simulink model "Crtl_Model_SS"  (R2015a)
settings: Solver=ode45  StartTime=0.0  StopTime=10.0  RelTol=1e-3
values from neighbouring files (symbols this model uses):
  ssDot = n4sid(data33, 3, 'DisturbanceModel', 'none', Options)    [Model_Centralizat.m]
  ssTHPS = ss(ssTHPS)    [Model_Centralizat.m]
  Te = t(2)-t(1)    [Models.m]    (also in shit_try.m = 0.003; simData_check.mat = 0.01; smth_new_025.m)
settings Model: Creator=Maria  LastModifiedBy=Maria

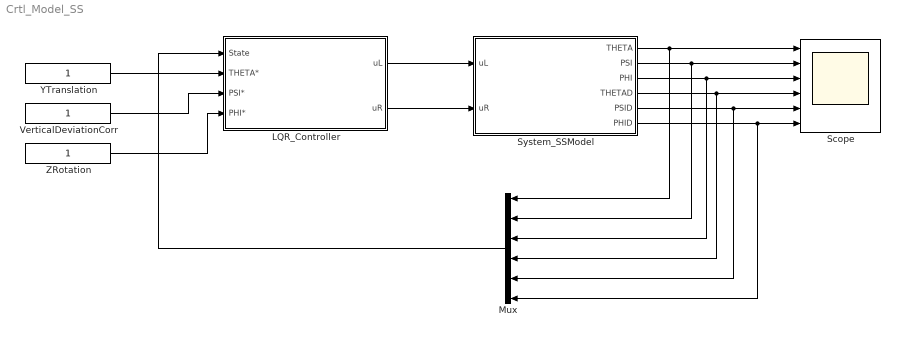
== system Crtl_Model_SS ==
  "LQR_Controller " : Subsystem
  Mux : Mux  Inputs=6
  Scope : Scope  NumInputPorts=6
      settings: YMin=-5~-5~-5~-5~-5~-5  YMax=5~5~5~5~5~5
  "System_SSModel " : Subsystem
  "VerticalDeviationCorr " : Constant
  "YTranslation " : Constant
  "ZRotation " : Constant
  wires:
  "System_SSModel "/2(PSI) -> Mux/2, Scope/2
  "System_SSModel "/1(THETA) -> Mux/1, Scope/1
  "System_SSModel "/3(PHI) -> Mux/3, Scope/3
  "System_SSModel "/5("PSID ") -> Mux/5, Scope/5
  "System_SSModel "/6(PHID) -> Mux/6, Scope/6
  "LQR_Controller "/1("uL ") -> "System_SSModel "/1(uL)
  "LQR_Controller "/2("uR ") -> "System_SSModel "/2("uR ")
  "YTranslation "/1 -> "LQR_Controller "/2(THETA*)
  "VerticalDeviationCorr "/1 -> "LQR_Controller "/3("PSI* ")
  "ZRotation "/1 -> "LQR_Controller "/4("PHI* ")
  "System_SSModel "/4("THETAD ") -> Mux/4, Scope/4
  Mux/1 -> "LQR_Controller "/1("State ")

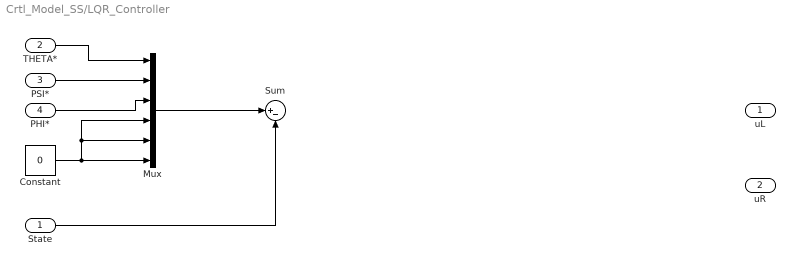
== system Crtl_Model_SS/LQR_Controller  ==
  "State " : Inport
  THETA* : Inport  Port=2
  "PSI* " : Inport  Port=3
  "PHI* " : Inport  Port=4
  Constant : Constant  Value=0
  Mux : Mux  Inputs=6
  Sum : Sum  Inputs=|+-
  "uL " : Outport
  "uR " : Outport  Port=2
  wires:
  THETA*/1 -> Mux/1
  "PSI* "/1 -> Mux/2
  "PHI* "/1 -> Mux/3
  Constant/1 -> Mux/5, Mux/4, Mux/6
  Mux/1 -> Sum/1
  "State "/1 -> Sum/2

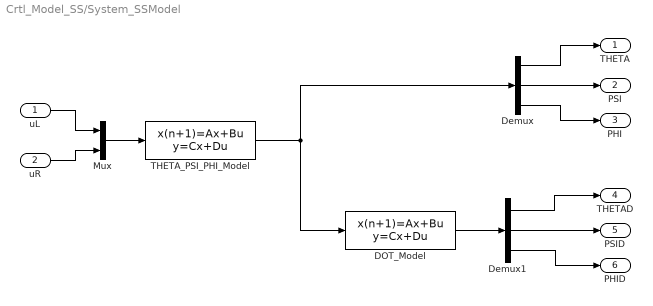
== system Crtl_Model_SS/System_SSModel  ==
  uL : Inport
  "uR " : Inport  Port=2
  DOT_Model : DiscreteStateSpace  A=[ssDot(1,1).a, ssDot(1,2).a, ssDot(1,3).a; ssDot(2,1).a, ssDot(2,2).a, ssDot(2,3).a; ssDot(3,1).a, ssDot(3,2).a, ssDot(3,3).a]  B=[ssDot(1,1).b, ssDot(1,2).b, ssDot(1,3).b; ssDot(2,1).b, ssDot(2,2).b, ssDot(2,3).b; ssDot(3,1).b, ssDot(3,2).b, ssDot(3,3).b]  C=[ssDot(1,1).c, ssDot(1,2).c, ssDot(1,3).c; ssDot(2,1).c, ssDot(2,2).c, ssDot(2,3).c; ssDot(3,1).c, ssDot(3,2).c, ssDot(3,3).c]  D=[ssDot(1,1).d, ssDot(1,2).d, ssDot(1,3).d; ssDot(2,1).d, ssDot(2,2).d, ssDot(2,3).d; ssDot(3,1).d, ssDot(3,2).d, ssDot(3,3).d]  SampleTime=Te
  Demux : Demux  Outputs=3
  Demux1 : Demux  Outputs=3
  Mux : Mux  Inputs=2
  THETA_PSI_PHI_Model : DiscreteStateSpace  A=[ssTHPS(1,1).a, ssTHPS(1,2).a; ssTHPS(2,1).a, ssTHPS(2,2).a]  B=[ssTHPS(1,1).b, ssTHPS(1,2).b; ssTHPS(2,1).b, ssTHPS(2,2).b]  C=[ssTHPS(1,1).c, ssTHPS(1,2).c; ssTHPS(2,1).c, ssTHPS(2,2).c]  D=[ssTHPS(1,1).d, ssTHPS(1,2).d; ssTHPS(2,1).d, ssTHPS(2,2).d]  SampleTime=Te
  THETA : Outport
  PSI : Outport  Port=2
  PHI : Outport  Port=3
  "THETAD " : Outport  Port=4
  "PSID " : Outport  Port=5
  PHID : Outport  Port=6
  wires:
  THETA_PSI_PHI_Model/1 -> Demux/1, DOT_Model/1
  Mux/1 -> THETA_PSI_PHI_Model/1
  uL/1 -> Mux/1
  "uR "/1 -> Mux/2
  DOT_Model/1 -> Demux1/1
  Demux/1 -> THETA/1
  Demux/2 -> PSI/1
  Demux/3 -> PHI/1
  Demux1/1 -> "THETAD "/1
  Demux1/2 -> "PSID "/1
  Demux1/3 -> PHID/1
